simulink model "exampleThermalNode"  (R2018b)
settings: Solver=ode45  StartTime=0.0  StopTime=3600  MaxStep=60  RelTol=1e-3  EnableMultiTasking=on
libraries: simulink x2, carnot x1
settings Model: Creator=drhf  LastModifiedBy=drhf
settings DataIOCC: LimitDataPoints=on  SaveFormat=Array  SignalLoggingSaveFormat=ModelDataLogs
settings OptimizationCC: ExpressionDepthLimit=2147483647  LifeSpan=inf
settings DebuggingCC: UnderspecifiedInitializationDetection=Classic  MergeDetectMultiDrivingBlocksExec=none  SolverPrmCheckMsg=warning  FcnCallInpInsideContextMsg=warning  StateNameClashWarn=warning  SFUnexpectedBacktrackingDiag=warning  SFNoUnconditionalDefaultTransitionDiag=warning  SFExecutionAtInitializationDiag=none
settings HardwareCC: ProdBitPerPointer=32  ProdBitPerSizeT=32  ProdBitPerPtrDiffT=32  ProdLargestAtomicFloat=None  ProdIntDivRoundTo=Undefined  ProdEndianess=Unspecified  ProdWordSize=32  ProdHWDeviceType=32-bit Generic
settings ModelReferenceCC: PropagateSignalLabelsOutOfModel=off
settings SFSimCC: SimUseLocalCustomCode=off
settings RTWCC: RTWUseLocalCustomCode=off
settings CodeAppCC: StateflowObjectComments=on
settings GRTTargetCC: TargetLangStandard=C89/C90 (ANSI)  GeneratePreprocessorConditionals=Disable all  CombineOutputUpdateFcns=off  GRTInterface=on
settings ConfigComp: CovMetricSettings=dw  CovHtmlReporting=on  CovSaveCumulativeToWorkspaceVar=on  CovSaveSingleToWorkspaceVar=on  CovExternalEMLEnable=off

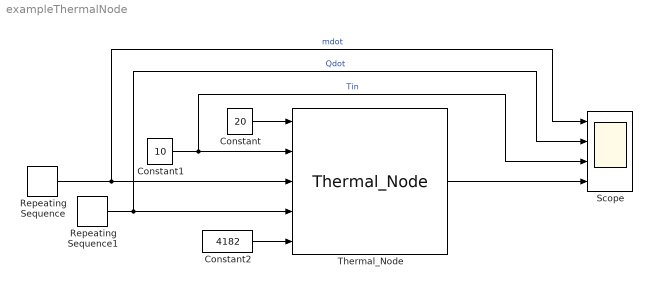
== system exampleThermalNode ==
  Constant : Constant  Value=20
  Constant1 : Constant  Value=10
  Constant2 : Constant  Value=4182
  Repeating Sequence : simulink/Sources/Repeating Sequence  rep_seq_t=[0 900 901 3601]  rep_seq_y=[0 0 0.1 0.1]
  Repeating Sequence1 : simulink/Sources/Repeating Sequence  rep_seq_t=[0 2000 2001 3601]  rep_seq_y=[0 0 5000 5000]
  Scope : Scope  NumInputPorts=4
  Thermal_Node : carnot/Basic/Thermal_Models/Thermal_Node  UA=10  mcp=3*4182
      settings: SourceProductName=Carnot
  wires:
  Thermal_Node/1 -> Scope/4
  Constant/1 -> Thermal_Node/1
  Constant1/1 -> Scope/3, Thermal_Node/2  "Tin"
  Repeating Sequence/1 -> Scope/1, Thermal_Node/3  "mdot"
  Repeating Sequence1/1 -> Thermal_Node/4, Scope/2  "Qdot"
  Constant2/1 -> Thermal_Node/5
